simulink model "sensor_dynamics"  (R2022a)
settings: Solver=ode45  StartTime=0.0  StopTime=12  RelTol=1e-6  AbsTol=1e-8
settings Model: Creator=HJL  LastModifiedBy=HJL

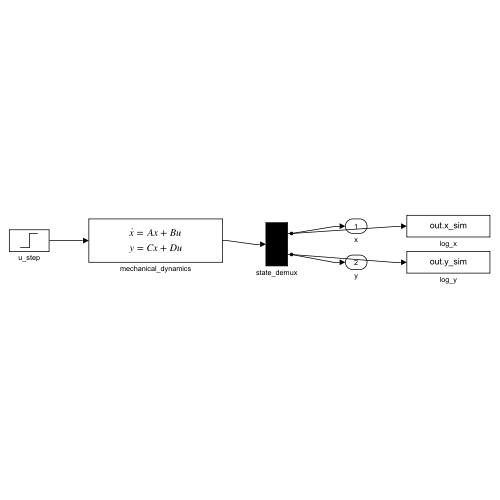
[thumbnail: Simulink's stored preview of the top-level diagram]
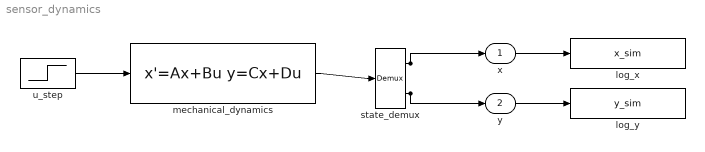
== system sensor_dynamics ==
  log_x : ToWorkspace  VariableName=x_sim  SaveFormat=Timeseries  SampleTime=-1
  log_y : ToWorkspace  VariableName=y_sim  SaveFormat=Timeseries  SampleTime=-1
  mechanical_dynamics : StateSpace  A=[0 1; -1.2 -0.2]  B=[0; 1]  C=[1 0; 0 1]  D=[0; 0]  InitialCondition=[0; 0]
  state_demux : Demux  Outputs=2
  u_step : Step  SampleTime=0
  x : Outport
  y : Outport  Port=2
  wires:
  u_step/1 -> mechanical_dynamics/1
  mechanical_dynamics/1 -> state_demux/1
  state_demux/1 -> x/1, log_x/1
  state_demux/2 -> y/1, log_y/1
